simulink model "gm_FSK_MODULATOR_HARDWARE_MODEL"  (R2024a)
settings: Solver=FixedStepDiscrete  StartTime=0.0  StopTime=3.5/B  FixedStep=1/fclk  RelTol=1e-3
undefined symbols (not defined in the file or in its folder): B, f0, fclk, XData
libraries: hdlsllib x1
(part 1 of 2)
settings Model: Creator=pc  LastModifiedBy=pc
settings OptimizationCC: BlockReduction=off  ConditionallyExecuteInputs=off  DefaultParameterBehavior=Inlined  OptimizeBlockIOStorage=off  EnhancedBackFolding=on  PassReuseOutputArgsAs=Individual arguments  OptimizeBlockOrder=speed  DifferentSizesBufferReuse=on  EfficientTunableParamExpr=on
settings DebuggingCC: InheritedTsInSrcMsg=none  ParameterTunabilityLossMsg=error
settings HardwareCC: TargetBitPerPointer=64  TargetBitPerSizeT=64  TargetBitPerPtrDiffT=64  TargetLongLongMode=on  TargetIntDivRoundTo=Zero  TargetEndianess=LittleEndian  TargetWordSize=64  TargetHWDeviceType=Generic->Custom  ProdEqTarget=off
settings SFSimCC: MATLABDynamicMemAlloc=off
settings RTWCC: Description=SystemVerilog DPI Component Generator  SystemTargetFile=systemverilog_dpi_ert.tlc  TemplateMakefile=systemverilog_dpi_ert_default_tmf
settings CodeAppCC: ForceParamTrailComments=on  IgnoreCustomStorageClasses=off  MaxIdLength=256  OperatorAnnotations=on  SimulinkDataObjDesc=on  SFDataObjDesc=on  InsertBlockDesc=on
settings DPIERTTargetCC: TargetFcnLib=ansi_tfl_table_tmw.mat  GenFloatMathFcnCalls=NOT IN USE  TargetLangStandard=C99 (ISO)  CodeReplacementLibrary=None  UtilityFuncGeneration=Auto  MultiwordTypeDef=System defined  MultiwordLength=2048  DynamicStringBufferSize=256  GenerateFullHeader=on  InferredTypesCompatibility=off  GenerateSampleERTMain=off  GenerateTestInterfaces=off  ModelReferenceCompliant=on  ParMdlRefBuildCompliant=on  CompOptLevelCompliant=off  ConcurrentExecutionCompliant=off  IncludeMdlTerminateFcn=on  CombineOutputUpdateFcns=off  CombineSignalStateStructs=on  GroupInternalDataByFunction=off  SuppressErrorStatus=off  IncludeFileDelimiter=Auto  ERTCustomFileBanners=on  SupportAbsoluteTime=on  LogVarNameModifier=rt_  MatFileLogging=off  CodeInterfacePackaging=Reusable function  PurelyIntegerCode=off  SupportNonFinite=on  SupportComplex=on  SupportContinuousTime=on  SupportNonInlinedSFcns=on  RemoveDisableFunc=off  RemoveResetFunc=on  SupportVariableSizeSignals=off  ParenthesesLevel=Nominal  CastingMode=Nominal  MATLABClassNameForMDSCustomization=Simulink.SoftwareTarget.TargetSpecificTriggerConfigurationBase  ModelStepFunctionPrototypeControlCompliant=on  CPPClassGenCompliant=off  AutosarCompliant=off  MDXCompliant=off  GRTInterface=off  GenerateAllocFcn=on  UseToolchainInfoCompliant=on  GenerateSharedConstants=on  CoderGroups=[]  AccessMethods=[]  LookupTableObjectStructAxisOrder=1,2,3,4,...  LUTObjectStructOrderExplicitValues=Size,Breakpoints,Table  LUTObjectStructOrderEvenSpacing=Size,Breakpoints,Table  ArrayLayout=Column-major  UnsupportedSFcnMsg=error  ERTHeaderFileRootName=$R$E  ERTSourceFileRootName=$R$E  ERTDataFileRootName=$R_data  InstructionSetFMA=off  OptimizeReductions=off  LogToMDFFile=off  GenerateASAP2=off  DSAsUniqueAccess=off  ExtMode=off  ExtModeTransport=0  ExtModeStaticAlloc=off  ExtModeAutomaticAllocSize=on  ExtModeMaxTrigDuration=10  ExtModeStaticAllocSize=1000000  ExtModeTesting=off  ExtModeMexFile=ext_comm  ExtModeIntrfLevel=Level1  InlinedParameterPlacement=NonHierarchical  TargetOS=BareBoardExample  MultiInstanceErrorCode=Error  RootIOFormat=Part of model data structure  RTWCAPISignals=on  RTWCAPIParams=off  RTWCAPIStates=off  RTWCAPIRootIO=off  ERTSrcFileBannerTemplate=ert_code_template.cgt  ERTHdrFileBannerTemplate=ert_code_template.cgt  ERTDataSrcFileTemplate=ert_code_template.cgt  ERTDataHdrFileTemplate=ert_code_template.cgt  ERTCustomFileTemplate=example_file_process.tlc  EnableDataOwnership=off  SignalDisplayLevel=10  ParamTuneLevel=10  GlobalDataDefinition=Auto  DataDefinitionFile=global.c  GlobalDataReference=Auto  ERTFilePackagingFormat=Modular  RateTransitionBlockCode=Inline  DataReferenceFile=global.h  PreserveExpressionOrder=off  PreserveIfCondition=off  ConvertIfToSwitch=on  PreserveExternInFcnDecls=on  PreserveStaticInFcnDecls=on  SuppressUnreachableDefaultCases=on  EnableSignedLeftShifts=on  EnableSignedRightShifts=on  ImplementImageWithCVMat=off  IndentStyle=K&R  IndentSize=2  NewlineStyle=Default  MaxLineWidth=80  EnableUserReplacementTypes=off  MaxIdInt64=MAX_int64_T  MinIdInt64=MIN_int64_T  MaxIdUint64=MAX_uint64_T  MaxIdInt32=MAX_int32_T  MinIdInt32=MIN_int32_T  MaxIdUint32=MAX_uint32_T  MaxIdInt16=MAX_int16_T  MinIdInt16=MIN_int16_T  MaxIdUint16=MAX_uint16_T  MaxIdInt8=MAX_int8_T  MinIdInt8=MIN_int8_T  MaxIdUint8=MAX_uint8_T  BooleanTrueId=true  BooleanFalseId=false  MemSecPackage=--- None ---  MemSecDataConstants=Default  MemSecDataIO=Default  MemSecDataInternal=Default  MemSecDataParameters=Default  MemSecFuncInitTerm=Default  MemSecFuncExecute=Default  MemSecFuncSharedUtil=Default  GroupConstants=Default  GroupRootInputs=Default  GroupRootOutputs=Default  GroupInternal=Default  GroupParameters=Default  GroupDataTransfer=Default  GroupSharedLocalDataStores=Default  GroupInstanceSpecificParameters=Default  GroupModelData=Default  ArrayContainerType=C-style array  DPICustomizeSystemVerilogCode=off  DPISystemVerilogTemplate=svdpi_event.vgt  DPIReportRunTimeError=off  DPIScalarizePorts=off  DPIRunTimeErrorSeverity=Fatal  DPIGenerateTestBench=off  DPITestBenchSimulator=Mentor Graphics Questasim  DPITestPointAccessFcnInterface=None  DPIFixedPointDataType=CompatibleCType  DPIPortConnection=Port list  DPICompositeDataType=Flattened  DPIComponentTemplateType=Sequential

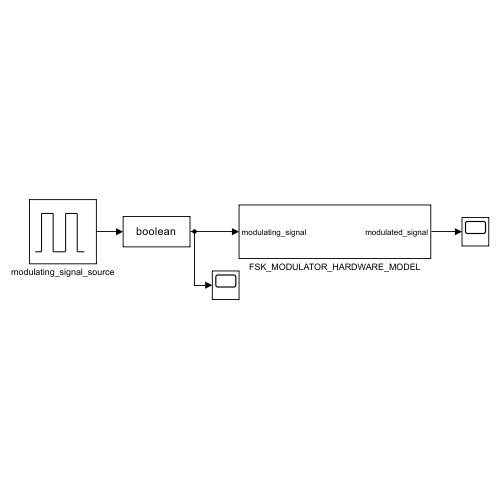
[thumbnail: Simulink's stored preview of the top-level diagram]
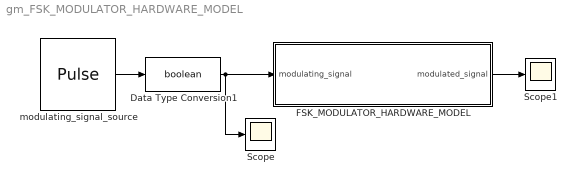
== system gm_FSK_MODULATOR_HARDWARE_MODEL ==
  Data Type Conversion1 : DataTypeConversion  OutDataTypeStr=boolean  SaturateOnIntegerOverflow=off  RndMeth=Floor
  FSK_MODULATOR_HARDWARE_MODEL : Subsystem
  Scope : Scope
  Scope1 : Scope
  modulating_signal_source : DiscretePulseGenerator  PulseType=Time based  Period=2/B  PulseWidth=50
  wires:
  FSK_MODULATOR_HARDWARE_MODEL/1(modulated_signal) -> Scope1/1
  modulating_signal_source/1 -> Data Type Conversion1/1
  Data Type Conversion1/1 -> Scope/1, FSK_MODULATOR_HARDWARE_MODEL/1(modulating_signal)

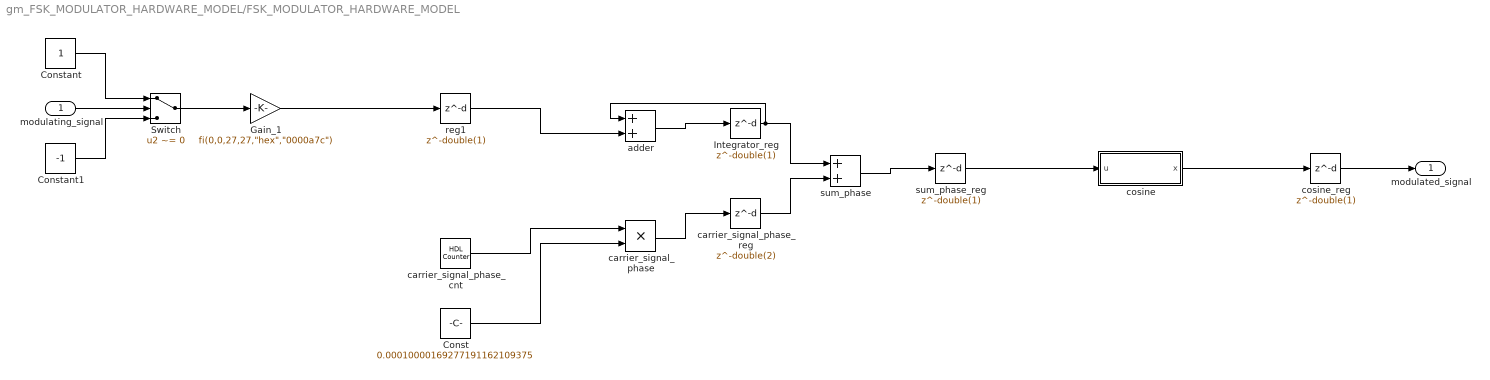
== system gm_FSK_MODULATOR_HARDWARE_MODEL/FSK_MODULATOR_HARDWARE_MODEL ==
  modulating_signal : Inport  OutDataTypeStr=boolean  PortDimensions=1  SampleTime=1e-08
  Const : Constant  Value=0.00010000169277191162109375  OutDataTypeStr=fixdt(0, 27, 27)  SampleTime=1e-08
  Constant : Constant  OutDataTypeStr=fixdt(1, 17, 15)  SampleTime=1e-08
  Constant1 : Constant  Value=-1  OutDataTypeStr=fixdt(1, 17, 15)  SampleTime=1e-08
  Gain_1 : Gain  Gain="fi(0,0,27,27,\"hex\",\"0000a7c\")"  ParamDataTypeStr=fixdt(0, 27, 27)  OutDataTypeStr=fixdt(1, 28, 27)  RndMeth=Round  SampleTime=1e-08
  Integrator_reg : Delay  DelayLength=double(1)  InitialCondition=0  SampleTime=1e-08
  Switch : Switch  Criteria=u2 ~= 0  Threshold=double(0)  OutDataTypeStr=fixdt(1, 17, 15)  SampleTime=1e-08  SaturateOnIntegerOverflow=off  InputSameDT=off
  adder : Sum  OutDataTypeStr=fixdt(1, 28, 27)  AccumDataTypeStr=fixdt(1, 28, 27)  SampleTime=1e-08
  carrier_signal_phase : Product  Inputs=**  OutDataTypeStr=fixdt(0, 28, 28)  SampleTime=1e-08
  carrier_signal_phase_cnt : hdlsllib/Sources/HDL Counter  CountType=Count limited  CountInit=0  CountStep=1  CountMax=fclk/f0  CountFromType=Initial value  CountFrom=0  CountResetPort=off  CountLoadPort=off  CountEnbPort=off  CountDirPort=off  CountHitOutputPort=off  CountDataType=Unsigned  CountWordLen=16  CountFracLen=0  CountSampTime=1/fclk
  carrier_signal_phase_reg : Delay  DelayLength=double(2)  InitialCondition=0  SampleTime=1e-08
  cosine : Subsystem  mask(Sine and Cosine HDL optimized block){OutputFormula=cos(2*pi*u), NumDataPoints=double(2048), TableDataTypeStr=fixdt(1,16,15), SimulateLUTROMDelay=on}
      mask prompts: OutputFormula "Simulink:masks:OutputFormula_MP"; NumDataPoints "HDLShared:hdlshared:CosineHDL_Npts"; TableDataTypeStr "Simulink:blkprm_prompts:TABLE_UNIFIEDDATATYPE"; SimulateLUTROMDelay "HDLShared:hdlshared:CosineHDL_SimulateLUTDelay"
      mask help: Sine and Cosine HDL optimized block using quarter wave symmetry, and HDL friendly settings.
      mask init:
      | NumDataPoints = double(2048);
      | OutputFormula = double(2);
      | SampleTime = double(-1);
      | SimulateLUTROMDelay = double(1);
      | TableDataTypeStr = fixdt(1,16,15);
      | curr_blk_name = 'FSK_MODULATOR_HARDWARE_MODEL/FSK_MODULATOR_HARDWARE_MODEL/cosine';
      | sys_name = 'FSK_MODULATOR_HARDWARE_MODEL/FSK_MODULATOR_HARDWARE_MODEL';
      mask Help: helpview([docroot '/hdlcoder/helptargets.map'],'SineAndCosineHDL_Optimized');
      mask TypeOptions OutputFormula: sin(2*pi*u) | cos(2*pi*u) | exp(j*2*pi*u) | sin(2*pi*u) and cos(2*pi*u)
      mask Display:
      | port_label('input',1,'u')
      | port_label('output',1,'cos(2*pi*u)')
      | xpos = 0.35;
      | yoffset = 0.5;
      | if ( SimulateLUTROMDelay )
      |   text(xpos,yoffset,'HDL (Z^{-1})','texmode','on')
      | else
      |    text(xpos,yoffset,'HDL')
      | end
  cosine_reg : Delay  DelayLength=double(1)  InitialCondition=0  SampleTime=1e-08
  reg1 : Delay  DelayLength=double(1)  InitialCondition=0  SampleTime=1e-08
  sum_phase : Sum  OutDataTypeStr=fixdt(1, 32, 28)  AccumDataTypeStr=fixdt(1, 29, 28)  SampleTime=1e-08
  sum_phase_reg : Delay  DelayLength=double(1)  InitialCondition=0  SampleTime=1e-08
  modulated_signal : Outport  SampleTime=1e-08
  wires:
  modulating_signal/1 -> Switch/2
  Const/1 -> carrier_signal_phase/2
  Constant/1 -> Switch/1
  Constant1/1 -> Switch/3
  Gain_1/1 -> reg1/1
  Switch/1 -> Gain_1/1
  carrier_signal_phase/1 -> carrier_signal_phase_reg/1
  carrier_signal_phase_cnt/1 -> carrier_signal_phase/1
  carrier_signal_phase_reg/1 -> sum_phase/2
  cosine/1(x) -> cosine_reg/1
  cosine_reg/1 -> modulated_signal/1
  reg1/1 -> adder/2
  sum_phase/1 -> sum_phase_reg/1
  sum_phase_reg/1 -> cosine/1(u)
  adder/1 -> Integrator_reg/1
  Integrator_reg/1 -> sum_phase/1, adder/1
